simulink library "custom_blocks"  (R2019b)
settings: Solver=VariableStepAuto  StartTime=0.0  StopTime=10.0  RelTol=1e-3
undefined symbols (not defined in the file): aMode, National_Instruments, PCIe, samp
libraries: simulink x25, powerlib_meascontrol x9, $bdroot x2, sldrtlib x1
(part 2 of 2)

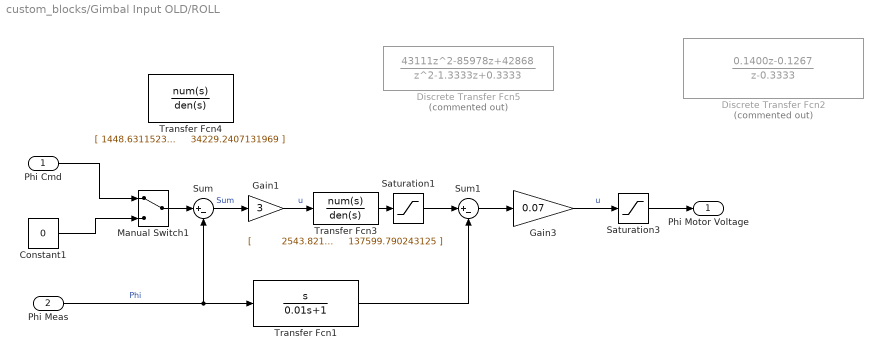
== system custom_blocks/Gimbal Input OLD/ROLL ==
  Phi Cmd : Inport
  Phi Meas : Inport  Port=2
  Constant1 : Constant  Value=0
  Discrete Transfer Fcn2 : DiscreteTransferFcn  Commented=on  Numerator="[0.1400   -0.1267]"  Denominator="[1   -0.3333]"  SampleTime=0.001
  Discrete Transfer Fcn5 : DiscreteTransferFcn  Commented=on  Numerator="[43111   -85978    42868]"  Denominator="[1   -1.3333    0.3333]"  SampleTime=0.001
  Gain1 : Gain  Gain=3
  Gain3 : Gain  Gain=0.07
  Manual Switch1 : ManualSwitch
  Saturation1 : Saturate  UpperLimit=600  LowerLimit=-600
  Saturation3 : Saturate  UpperLimit=10  LowerLimit=-10
  Sum : Sum  Inputs=|+-
  Sum1 : Sum  Inputs=|+-
  Transfer Fcn1 : TransferFcn  Numerator=[1 0]  Denominator=[0.01 1]
  Transfer Fcn3 : TransferFcn  Numerator=|  Denominator=|
      Numerator=|
      | [          2543.82143144429          511903.158690718          32769948.6587151
      | ]
      Denominator=|
      | [                         1          736.044036108538          137599.790243125
      | ]
  Transfer Fcn4 : TransferFcn  Numerator="[ 1448.63115231632          112858.338645866          13691696.2852788]"  Denominator=|
      | [                         1          369.516093474425          34229.2407131969
      | ]
  Phi Motor Voltage : Outport
  wires:
  Gain1/1 -> Transfer Fcn3/1  "u"
  Saturation1/1 -> Sum1/1
  Transfer Fcn3/1 -> Saturation1/1
  Sum/1 -> Gain1/1  "Sum"
  Saturation3/1 -> Phi Motor Voltage/1
  Gain3/1 -> Saturation3/1  "u"
  Transfer Fcn1/1 -> Sum1/2
  Phi Cmd/1 -> Manual Switch1/1
  Constant1/1 -> Manual Switch1/2
  Manual Switch1/1 -> Sum/1
  Sum1/1 -> Gain3/1
  Phi Meas/1 -> Sum/2, Transfer Fcn1/1  "Phi"

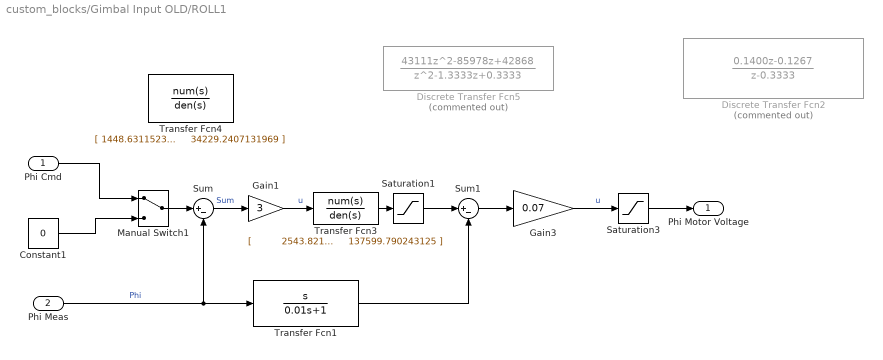
== system custom_blocks/Gimbal Input OLD/ROLL1 ==
  Phi Cmd : Inport
  Phi Meas : Inport  Port=2
  Constant1 : Constant  Value=0
  Discrete Transfer Fcn2 : DiscreteTransferFcn  Commented=on  Numerator="[0.1400   -0.1267]"  Denominator="[1   -0.3333]"  SampleTime=0.001
  Discrete Transfer Fcn5 : DiscreteTransferFcn  Commented=on  Numerator="[43111   -85978    42868]"  Denominator="[1   -1.3333    0.3333]"  SampleTime=0.001
  Gain1 : Gain  Gain=3
  Gain3 : Gain  Gain=0.07
  Manual Switch1 : ManualSwitch
  Saturation1 : Saturate  UpperLimit=600  LowerLimit=-600
  Saturation3 : Saturate  UpperLimit=10  LowerLimit=-10
  Sum : Sum  Inputs=|+-
  Sum1 : Sum  Inputs=|+-
  Transfer Fcn1 : TransferFcn  Numerator=[1 0]  Denominator=[0.01 1]
  Transfer Fcn3 : TransferFcn  Numerator=|  Denominator=|
      Numerator=|
      | [          2543.82143144429          511903.158690718          32769948.6587151
      | ]
      Denominator=|
      | [                         1          736.044036108538          137599.790243125
      | ]
  Transfer Fcn4 : TransferFcn  Numerator="[ 1448.63115231632          112858.338645866          13691696.2852788]"  Denominator=|
      | [                         1          369.516093474425          34229.2407131969
      | ]
  Phi Motor Voltage : Outport
  wires:
  Phi Meas/1 -> Transfer Fcn1/1, Sum/2  "Phi"
  Sum1/1 -> Gain3/1
  Manual Switch1/1 -> Sum/1
  Constant1/1 -> Manual Switch1/2
  Phi Cmd/1 -> Manual Switch1/1
  Transfer Fcn1/1 -> Sum1/2
  Gain3/1 -> Saturation3/1  "u"
  Saturation3/1 -> Phi Motor Voltage/1
  Sum/1 -> Gain1/1  "Sum"
  Transfer Fcn3/1 -> Saturation1/1
  Saturation1/1 -> Sum1/1
  Gain1/1 -> Transfer Fcn3/1  "u"

== system custom_blocks/Gimbal Input OLD/YAW ==
  Psi Cmd : Inport
  Psi Meas : Inport  Port=2
  Cin : TransferFcn  Numerator=2.9192*[1 53.87]  Denominator=[1 200]
  Constant1 : Constant  Value=180
  Gain : Gain  Gain=0.1
  Manual Switch1 : ManualSwitch
  Saturation2 : Saturate  UpperLimit=100  LowerLimit=-100
  Sum : Sum  Inputs=|+-
  Sum1 : Sum  Inputs=|+-
  Transfer Fcn1 : TransferFcn  Numerator=|  Denominator=|
      Numerator=|
      | [          1048.88683783117          153388.518090953          10291300.4472415
      | ]
      Denominator=|
      | [                         1          457.625701221523           57405.478732949
      | ]
  Zero-Order Hold3 : ZeroOrderHold  SampleTime=0.01
  diff : TransferFcn  Numerator=[1 0]  Denominator=[0.01 1]
  error1 : Scope
  Psi Motor Voltage : Outport
  wires:
  Sum1/1 -> Cin/1
  Gain/1 -> Transfer Fcn1/1
  Zero-Order Hold3/1 -> Psi Motor Voltage/1
  Cin/1 -> Zero-Order Hold3/1  "Phi"
  Transfer Fcn1/1 -> Saturation2/1
  Sum/1 -> Gain/1
  Constant1/1 -> Manual Switch1/2
  Psi Cmd/1 -> Manual Switch1/1
  Manual Switch1/1 -> Sum/1
  Saturation2/1 -> Sum1/1
  Psi Meas/1 -> Sum/2, diff/1
  diff/1 -> Sum1/2, error1/1  "Phi dot"

== system custom_blocks/Gimbal Input OLD/YAW1 ==
  Psi Cmd : Inport
  Psi Meas : Inport  Port=2
  Cin : TransferFcn  Numerator=2.9192*[1 53.87]  Denominator=[1 200]
  Constant1 : Constant  Value=180
  Gain : Gain  Gain=0.1
  Manual Switch1 : ManualSwitch
  Saturation2 : Saturate  UpperLimit=100  LowerLimit=-100
  Sum : Sum  Inputs=|+-
  Sum1 : Sum  Inputs=|+-
  Transfer Fcn1 : TransferFcn  Numerator=|  Denominator=|
      Numerator=|
      | [          1048.88683783117          153388.518090953          10291300.4472415
      | ]
      Denominator=|
      | [                         1          457.625701221523           57405.478732949
      | ]
  Zero-Order Hold3 : ZeroOrderHold  SampleTime=0.01
  diff : TransferFcn  Numerator=[1 0]  Denominator=[0.01 1]
  error1 : Scope
  Psi Motor Voltage : Outport
  wires:
  diff/1 -> error1/1, Sum1/2  "Phi dot"
  Psi Meas/1 -> diff/1, Sum/2
  Saturation2/1 -> Sum1/1
  Manual Switch1/1 -> Sum/1
  Psi Cmd/1 -> Manual Switch1/1
  Constant1/1 -> Manual Switch1/2
  Sum/1 -> Gain/1
  Transfer Fcn1/1 -> Saturation2/1
  Cin/1 -> Zero-Order Hold3/1  "Phi"
  Zero-Order Hold3/1 -> Psi Motor Voltage/1
  Gain/1 -> Transfer Fcn1/1
  Sum1/1 -> Cin/1

== system custom_blocks/Gimbal Motors/Phi deadzone ==
  Phi U : Inport
  Gain1 : Gain  Gain=0.32
  Sign : Signum
  Sum : Sum  Inputs=|++
  Phi V : Outport
  wires:
  Sum/1 -> Phi V/1
  Sign/1 -> Gain1/1
  Phi U/1 -> Sum/1, Sign/1
  Gain1/1 -> Sum/2

== system custom_blocks/Gimbal Motors/Subsystem ==
  Theta U : Inport
  Gain : Gain  Gain=-1
  Gain1 : Gain  Gain=0.098
  Sign : Signum
  Sum : Sum  Inputs=|++
  Theta V : Outport
  wires:
  Sign/1 -> Gain1/1
  Gain1/1 -> Sum/2
  Sum/1 -> Theta V/1
  Theta U/1 -> Gain/1
  Gain/1 -> Sum/1, Sign/1

== system custom_blocks/Gimbal Motors/Subsystem1 ==
  Psi U : Inport
  Gain1 : Gain  Gain=0.217
  Sign : Signum
  Sum : Sum  Inputs=|++
  Psi V : Outport
  wires:
  Sign/1 -> Gain1/1
  Gain1/1 -> Sum/2
  Sum/1 -> Psi V/1
  Psi U/1 -> Sum/1, Sign/1

== system custom_blocks/Index Locations/Triggered Subsystem ==
  In1 : Inport
  Trigger : TriggerPort  VariantControl=Variant
  Out1 : Outport  InitialOutput=-1
  wires:
  In1/1 -> Out1/1

== system custom_blocks/Index Locations/Triggered Subsystem1 ==
  In1 : Inport
  Trigger : TriggerPort  VariantControl=Variant
  Out1 : Outport  InitialOutput=-1
  wires:
  In1/1 -> Out1/1

== system custom_blocks/Index Locations/Triggered Subsystem2 ==
  In1 : Inport
  Trigger : TriggerPort  VariantControl=Variant
  Out1 : Outport  InitialOutput=-1
  wires:
  In1/1 -> Out1/1

== system custom_blocks/Index Locations OLD/Triggered Subsystem ==
  In1 : Inport
  Trigger : TriggerPort  VariantControl=Variant
  Out1 : Outport  InitialOutput=-1
  wires:
  In1/1 -> Out1/1

== system custom_blocks/Index Locations OLD/Triggered Subsystem1 ==
  In1 : Inport
  Trigger : TriggerPort  VariantControl=Variant
  Out1 : Outport  InitialOutput=-1
  wires:
  In1/1 -> Out1/1

== system custom_blocks/Index Locations OLD/Triggered Subsystem2 ==
  In1 : Inport
  Trigger : TriggerPort  VariantControl=Variant
  Out1 : Outport  InitialOutput=-1
  wires:
  In1/1 -> Out1/1

== system custom_blocks/Toggle Attitude Reached/Toggle ==
  Trigger : TriggerPort  VariantControl=Variant
  One : Constant  OutDataTypeStr=Inherit: Inherit via back propagation
  Out1 : Outport  InitialOutput=0
  wires:
  One/1 -> Out1/1

== system custom_blocks/Toggle Attitude Reached/primitive_differentation ==
  angle : Inport
  Delay : Delay  SampleTime=0.01
  Gain : Gain  Gain=1/0.02
  Subtract3 : Sum  Inputs=+-
  Zero-Order Hold3 : ZeroOrderHold  SampleTime=0.01
  angle dot : Outport
  wires:
  Gain/1 -> Zero-Order Hold3/1
  Zero-Order Hold3/1 -> angle dot/1
  Delay/1 -> Subtract3/2
  angle/1 -> Delay/1, Subtract3/1
  Subtract3/1 -> Gain/1
